simulink model "clark_park"  (R2024a)
settings: Solver=ode4  StartTime=0.0  StopTime=5  FixedStep=0.01  RelTol=1e-3
model workspace (MAT data in the model file):
  k = 0.666666666667
  w = 6.28318530718
settings Model: Creator=10472  LastModifiedBy=Administrator
settings SolverCC: AlgebraicLoopSolver=TrustRegion
settings DebuggingCC: UnconnectedInputMsg=warning  UnconnectedOutputMsg=warning  UnconnectedLineMsg=warning
settings ModelReferenceCC: EnableRefExpFcnMdlSchedulingChecks=on
settings RTWCC: GPUComputeCapability=3.5  DLArmComputeVersion=19.05

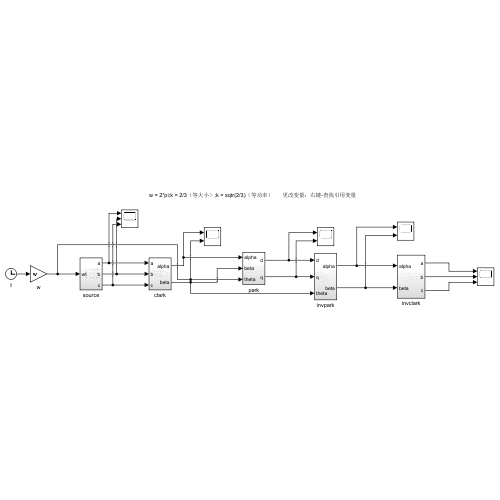
[thumbnail: Simulink's stored preview of the top-level diagram]
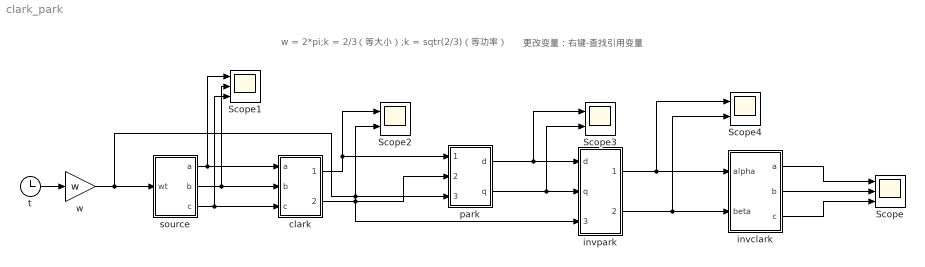
== system clark_park ==
  note: 更改变量：右键-查找引用变量
  note: w = 2*pi;k = 2/3（等大小）;k = sqtr(2/3)（等功率）
  Scope : Scope  NumInputPorts=3
  Scope1 : Scope  NumInputPorts=3
  Scope2 : Scope  NumInputPorts=2
  Scope3 : Scope  NumInputPorts=2
  Scope4 : Scope  NumInputPorts=2
  clark : Subsystem
  invclark : Subsystem
  invpark : Subsystem
  park : Subsystem
  source : Subsystem
  t : Clock
  w : Gain  Gain=w
  wires:
  t/1 -> w/1
  w/1 -> invpark/3(theta), park/3(theta), source/1(wt)
  source/1(a) -> Scope1/1, clark/1(a)
  source/2(b) -> Scope1/2, clark/2(b)
  source/3(c) -> clark/3(c), Scope1/3
  clark/1(alpha) -> park/1(alpha), Scope2/1
  clark/2(beta) -> park/2(beta), Scope2/2
  invclark/1(a) -> Scope/1
  invclark/2(b) -> Scope/2
  invclark/3(c) -> Scope/3
  park/1(d) -> Scope3/1, invpark/1(d)
  park/2(q) -> Scope3/2, invpark/2(q)
  invpark/1(alpha) -> Scope4/1, invclark/1(alpha)
  invpark/2(beta) -> Scope4/2, invclark/2(beta)

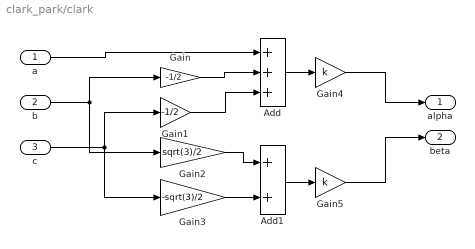
== system clark_park/clark ==
  a : Inport
  b : Inport  Port=2
  c : Inport  Port=3
  Add : Sum  Inputs=+++
  Add1 : Sum
  Gain : Gain  Gain=-1/2
  Gain1 : Gain  Gain=-1/2
  Gain2 : Gain  Gain=sqrt(3)/2
  Gain3 : Gain  Gain=-sqrt(3)/2
  Gain4 : Gain  Gain=k
  Gain5 : Gain  Gain=k
  alpha : Outport
  beta : Outport  Port=2
  wires:
  Gain/1 -> Add/2
  Gain1/1 -> Add/3
  Add1/1 -> Gain5/1
  b/1 -> Gain2/1, Gain/1
  Add/1 -> Gain4/1
  Gain3/1 -> Add1/2
  Gain4/1 -> alpha/1
  c/1 -> Gain1/1, Gain3/1
  Gain2/1 -> Add1/1
  a/1 -> Add/1
  Gain5/1 -> beta/1

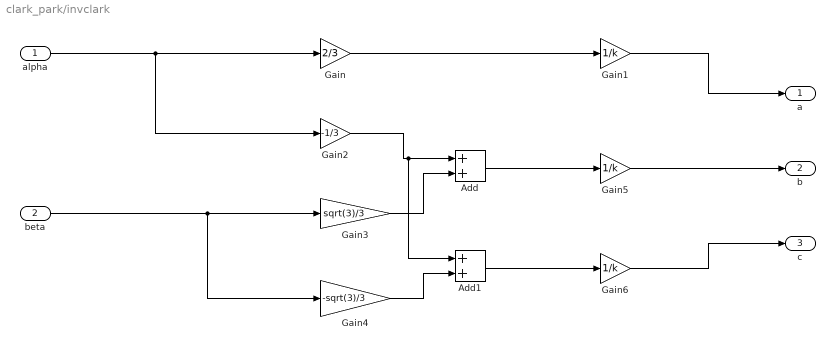
== system clark_park/invclark ==
  alpha : Inport
  beta : Inport  Port=2
  Add : Sum
  Add1 : Sum
  Gain : Gain  Gain=2/3
  Gain1 : Gain  Gain=1/k
  Gain2 : Gain  Gain=-1/3
  Gain3 : Gain  Gain=sqrt(3)/3
  Gain4 : Gain  Gain=-sqrt(3)/3
  Gain5 : Gain  Gain=1/k
  Gain6 : Gain  Gain=1/k
  a : Outport
  b : Outport  Port=2
  c : Outport  Port=3
  wires:
  Add1/1 -> Gain6/1
  Gain5/1 -> b/1
  beta/1 -> Gain4/1, Gain3/1
  Gain1/1 -> a/1
  Gain/1 -> Gain1/1
  Add/1 -> Gain5/1
  Gain6/1 -> c/1
  Gain4/1 -> Add1/2
  Gain2/1 -> Add1/1, Add/1
  alpha/1 -> Gain2/1, Gain/1
  Gain3/1 -> Add/2

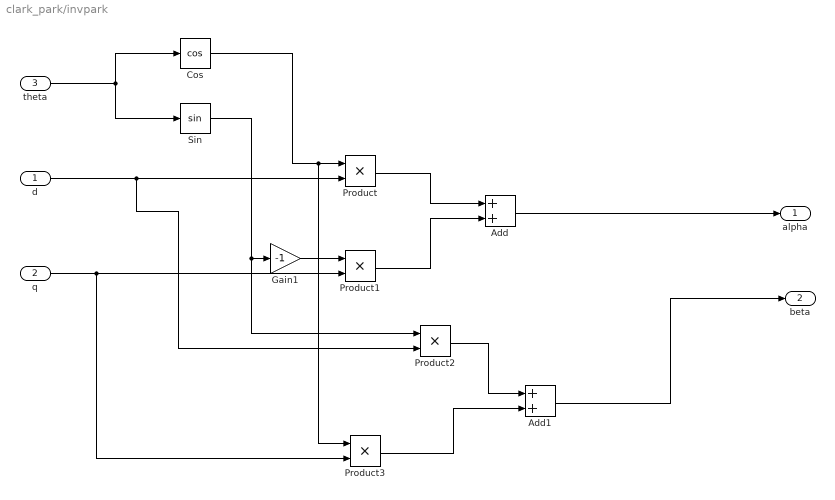
== system clark_park/invpark ==
  d : Inport
  q : Inport  Port=2
  theta : Inport  Port=3
  Add : Sum
  Add1 : Sum
  Cos : Trigonometry  Operator=cos
  Gain1 : Gain  Gain=-1
  Product{,1..3} (4 alike) : Product
  Sin : Trigonometry
  alpha : Outport
  beta : Outport  Port=2
  wires:
  Add1/1 -> beta/1
  Product3/1 -> Add1/2
  Product2/1 -> Add1/1
  Sin/1 -> Product2/1, Gain1/1
  Add/1 -> alpha/1
  Product1/1 -> Add/2
  Product/1 -> Add/1
  q/1 -> Product1/2, Product3/2
  Cos/1 -> Product/1, Product3/1
  d/1 -> Product/2, Product2/2
  theta/1 -> Cos/1, Sin/1
  Gain1/1 -> Product1/1

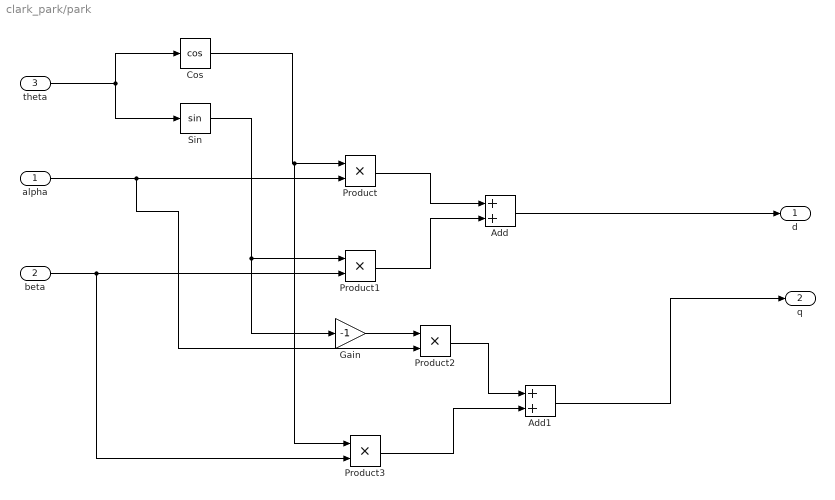
== system clark_park/park ==
  alpha : Inport
  beta : Inport  Port=2
  theta : Inport  Port=3
  Add : Sum
  Add1 : Sum
  Cos : Trigonometry  Operator=cos
  Gain : Gain  Gain=-1
  Product{,1..3} (4 alike) : Product
  Sin : Trigonometry
  d : Outport
  q : Outport  Port=2
  wires:
  theta/1 -> Sin/1, Cos/1
  alpha/1 -> Product2/2, Product/2
  Cos/1 -> Product3/1, Product/1
  beta/1 -> Product3/2, Product1/2
  Sin/1 -> Gain/1, Product1/1
  Product/1 -> Add/1
  Product1/1 -> Add/2
  Add/1 -> d/1
  Gain/1 -> Product2/1
  Product2/1 -> Add1/1
  Product3/1 -> Add1/2
  Add1/1 -> q/1

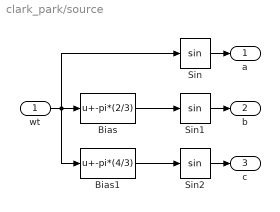
== system clark_park/source ==
  wt : Inport
  Bias : Bias  Bias=-pi*(2/3)  SaturateOnIntegerOverflow=off
  Bias1 : Bias  Bias=-pi*(4/3)  SaturateOnIntegerOverflow=off
  Sin : Trigonometry
  Sin1 : Trigonometry
  Sin2 : Trigonometry
  a : Outport
  b : Outport  Port=2
  c : Outport  Port=3
  wires:
  wt/1 -> Bias1/1, Sin/1, Bias/1
  Bias/1 -> Sin1/1
  Sin1/1 -> b/1
  Bias1/1 -> Sin2/1
  Sin2/1 -> c/1
  Sin/1 -> a/1
